simulink model "BlockDprob2c"  (R2017a)
settings: Solver=VariableStepAuto  StartTime=0.0  StopTime=230.0  RelTol=1e-3
values from neighbouring files (symbols this model uses):
  a1 = 2.87    [T_2d.m]    (also in controller.m; run_task_2e.m)
  a2 = -0.65    [T_2d.m]    (also in controller.m; run_task_2e.m)
  d = 2    [T_2d.m]    (also in run_task_2e.m)
  g = 9.81    [T_2d.m]    (also in run_task_2e.m)
  k_d_phi = f_kd(zp, wp)    [T_2d.m]    (also in run_task_2e.m)
  k_i_chi = V_g/g * wx^2    [T_2d.m]    (also in run_task_2e.m)
  k_i_phi = 0    [T_2d.m]    (also in run_task_2e.m)
  k_p_chi = V_g/g * 2*zx*wx    [T_2d.m]    (also in run_task_2e.m)
  k_p_phi = -5/3    (= -1.66666666667)    [T_2d.m]    (also in run_task_2e.m)
  V_g = 637/3.6    (= 176.944444444)    [T_2d.m]    (also in run_task_2e.m)
libraries: simulink_extras x4
settings Model: Creator=helene  LastModifiedBy=jljoberg

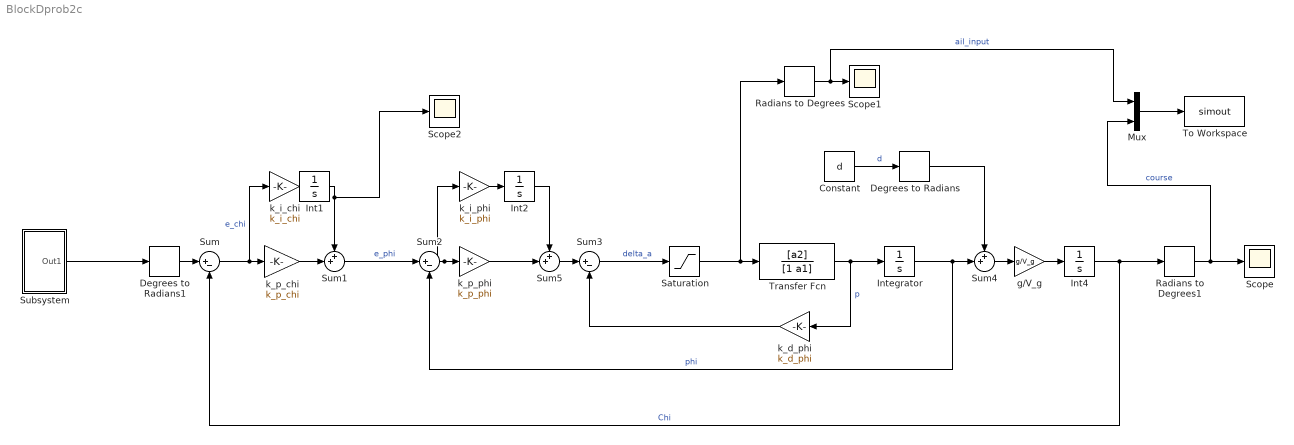
== system BlockDprob2c ==
  Constant : Constant  Value=d
  Degrees to Radians : simulink_extras/Transformations/Degrees to Radians
  Degrees to Radians1 : simulink_extras/Transformations/Degrees to Radians
  "Int1 " : Integrator  LimitOutput=on  UpperSaturationLimit=0.15  LowerSaturationLimit=-0.15
  "Int2 " : Integrator
  Int4 : Integrator
  Integrator : Integrator
  Mux : Mux  Inputs=2
  Radians to Degrees : simulink_extras/Transformations/Radians to Degrees
  Radians to Degrees1 : simulink_extras/Transformations/Radians to Degrees
  Saturation : Saturate  UpperLimit=25*deg2rad  LowerLimit=-25*deg2rad
  Scope : Scope
  Scope1 : Scope
  Scope2 : Scope
  Subsystem : Subsystem
  Sum : Sum  Inputs=|+-
  Sum1 : Sum  Inputs=++|
  Sum2 : Sum  Inputs=|+-
  Sum3 : Sum  Inputs=|+-
  Sum4 : Sum  Inputs=++|
  Sum5 : Sum  Inputs=++|
  To Workspace : ToWorkspace  VariableName=simout  SaveFormat=Timeseries  SampleTime=-1
  Transfer Fcn : TransferFcn  Numerator=[a2]  Denominator=[1 a1]
  g/V_g : Gain  Gain=g/V_g
  k_d_phi : Gain  Gain=k_d_phi
  k_i_chi : Gain  Gain=k_i_chi
  k_i_phi : Gain  Gain=k_i_phi
  k_p_chi : Gain  Gain=k_p_chi
  "k_p_phi " : Gain  Gain=k_p_phi
  wires:
  k_p_chi/1 -> Sum1/2
  Sum/1 -> k_i_chi/1, k_p_chi/1  "e_chi"
  k_i_chi/1 -> "Int1 "/1
  Sum2/1 -> k_i_phi/1, "k_p_phi "/1
  k_i_phi/1 -> "Int2 "/1
  "Int2 "/1 -> Sum5/1
  "k_p_phi "/1 -> Sum5/2
  Sum5/1 -> Sum3/1
  Transfer Fcn/1 -> Integrator/1, k_d_phi/1  "p"
  k_d_phi/1 -> Sum3/2
  Sum3/1 -> Saturation/1  "delta_a"
  Integrator/1 -> Sum2/2, Sum4/2  "phi"
  Sum4/1 -> g/V_g/1
  Int4/1 -> Radians to Degrees1/1, Sum/2  "Chi"
  Constant/1 -> Degrees to Radians/1  "d"
  g/V_g/1 -> Int4/1
  Radians to Degrees1/1 -> Mux/2, Scope/1  "course"
  Radians to Degrees/1 -> Mux/1, Scope1/1  "ail_input"
  Sum1/1 -> Sum2/1  "e_phi"
  Degrees to Radians/1 -> Sum4/1
  Degrees to Radians1/1 -> Sum/1
  Saturation/1 -> Radians to Degrees/1, Transfer Fcn/1
  "Int1 "/1 -> Scope2/1, Sum1/1
  Mux/1 -> To Workspace/1
  Subsystem/1(Out1) -> Degrees to Radians1/1

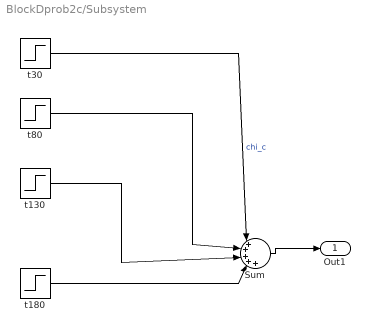
== system BlockDprob2c/Subsystem ==
  Sum : Sum  Inputs=|+++++
  t130 : Step  Time=130  After=-15  SampleTime=0
  t180 : Step  Time=180  After=-10  SampleTime=0
  t30 : Step  Time=30  After=15  SampleTime=0
  "t80 " : Step  Time=80  After=10  SampleTime=0
  Out1 : Outport
  wires:
  Sum/1 -> Out1/1
  t30/1 -> Sum/1  "chi_c"
  "t80 "/1 -> Sum/2
  t130/1 -> Sum/3
  t180/1 -> Sum/4
